simulink library "prakt4_1"  (R2025b)
settings: Solver=VariableStepAuto  StartTime=0.0  StopTime=10.0  RelTol=1e-3
settings Model: Creator=danieltchoudovski  LastModifiedBy=danieltchoudovski

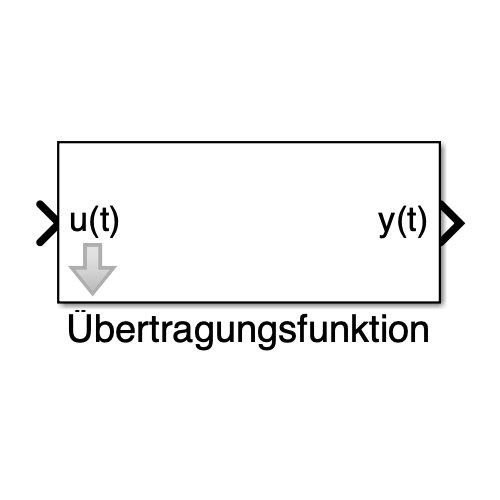
[thumbnail: Simulink's stored preview of the top-level diagram]
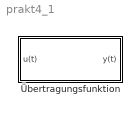
== system prakt4_1 ==
  Übertragungsfunktion : Subsystem  mask{T=1, Kp=1}
      mask prompts: T "Zeitkonst"; Kp "verstärkungsfaktor"

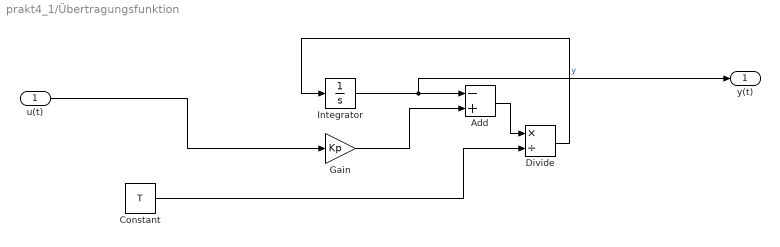
== system prakt4_1/Übertragungsfunktion ==
  u(t) : Inport
  Add : Sum  Inputs=-+
  Constant : Constant  Value=T
  Divide : Product  Inputs=*/
  Gain : Gain  Gain=Kp
  Integrator : Integrator
  y(t) : Outport
  wires:
  Add/1 -> Divide/1
  u(t)/1 -> Gain/1
  Divide/1 -> Integrator/1
  Constant/1 -> Divide/2
  Gain/1 -> Add/2
  Integrator/1 -> Add/1, y(t)/1  "y"
